simulink model "ejercicio_B"  (R2018a)
settings: Solver=VariableStepAuto  StartTime=0.0  StopTime=10.0  RelTol=1e-3
settings Model: Creator=Jorja_000  LastModifiedBy=Jorja_000

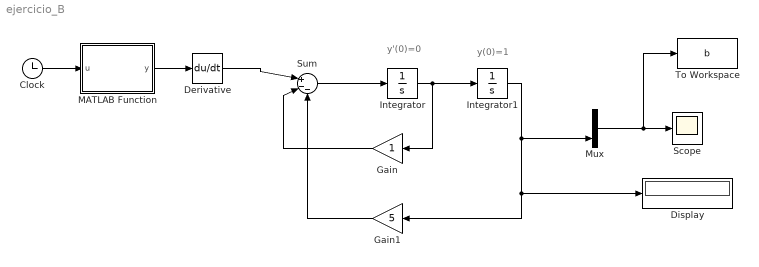
== system ejercicio_B ==
  note: y(0)=1
  note: y'(0)=0
  Clock : Clock
  Derivative : Derivative
  Display : Display
  Gain : Gain
  Gain1 : Gain  Gain=5
  Integrator : Integrator
  Integrator1 : Integrator  InitialCondition=1
  MATLAB Function : MATLAB Function  TreatAsAtomicUnit=on
  Mux : Mux  Inputs=2
  Scope : Scope
  Sum : Sum  Inputs=|+--
  To Workspace : ToWorkspace  VariableName=b  SaveFormat=Timeseries  SampleTime=-1
  wires:
  Sum/1 -> Integrator/1
  Clock/1 -> MATLAB Function/1(u)
  Mux/1 -> To Workspace/1, Scope/1
  Gain/1 -> Sum/2
  Integrator1/1 -> Mux/2, Display/1, Gain1/1
  Integrator/1 -> Gain/1, Integrator1/1
  Gain1/1 -> Sum/3
  MATLAB Function/1(y) -> Derivative/1
  Derivative/1 -> Sum/1

== matlab function ejercicio_B/MATLAB Function ==
  data: u input; y output
function y = fcn(u)

if(u>=0)
    y=1;
else
    y=0;
end
